simulink model "HoppingRobotModel"  (R2019b)
settings: Solver=VariableStepAuto  StartTime=0.0  StopTime=10.0  RelTol=1e-3
undefined symbols (not defined in the file): g, I1, ini_theta_1, ini_thetad_1, M2, r1, r2
settings Model: Creator=fabia  LastModifiedBy=fabia

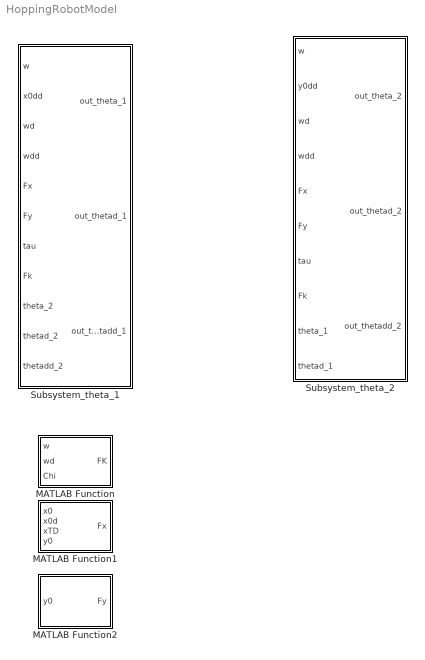
== system HoppingRobotModel ==
  MATLAB Function : MATLAB Function  TreatAsAtomicUnit=on
  MATLAB Function1 : MATLAB Function  TreatAsAtomicUnit=on
  MATLAB Function2 : MATLAB Function  TreatAsAtomicUnit=on
  Subsystem_theta_1 : Subsystem
  Subsystem_theta_2 : Subsystem

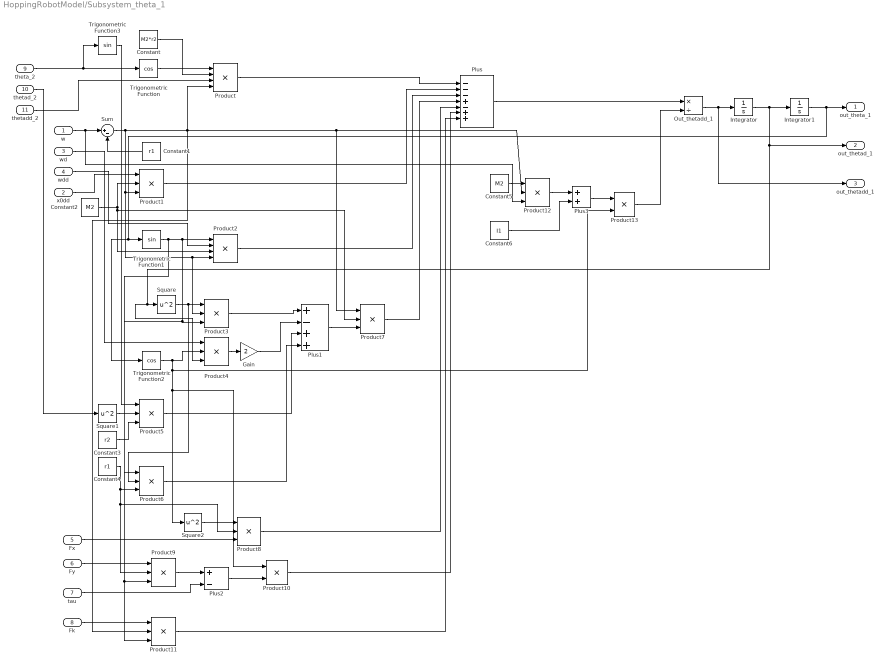
== system HoppingRobotModel/Subsystem_theta_1 ==
  w : Inport
  x0dd : Inport  Port=2
  wd : Inport  Port=3
  wdd : Inport  Port=4
  Fx : Inport  Port=5
  Fy : Inport  Port=6
  tau : Inport  Port=7
  Fk : Inport  Port=8
  theta_2 : Inport  Port=9
  thetad_2 : Inport  Port=10
  thetadd_2 : Inport  Port=11
  Constant : Constant  Value=M2*r2
  Constant1 : Constant  Value=r1
  Constant2 : Constant  Value=M2
  Constant3 : Constant  Value=r2
  Constant4 : Constant  Value=r1
  Constant5 : Constant  Value=M2
  Constant6 : Constant  Value=I1
  Gain : Gain  Gain=2
  Integrator : Integrator  InitialCondition=ini_thetad_1
  Integrator1 : Integrator  InitialCondition=ini_theta_1
  Out_thetadd_1 : Product  Inputs=*/
  Plus : Sum  Inputs=---+-++
  Plus1 : Sum  Inputs=+-++
  Plus2 : Sum  Inputs=+-
  Plus3 : Sum
  Product : Product  Inputs=4
  Product{1,3..9,11..12} (10 alike) : Product  Inputs=3
  Product10 : Product
  Product13 : Product
  Product2 : Product  Inputs=4
  Square : Math  Operator=square  SignedPower=off  SaturateOnIntegerOverflow=on
  Square1 : Math  Operator=square  SignedPower=off  SaturateOnIntegerOverflow=on
  Square2 : Math  Operator=square  SignedPower=off  SaturateOnIntegerOverflow=on
  Sum : Sum  Inputs=|+-
  Trigonometric Function : Trigonometry  Operator=cos
  Trigonometric Function1 : Trigonometry
  Trigonometric Function2 : Trigonometry  Operator=cos
  Trigonometric Function3 : Trigonometry
  out_theta_1 : Outport
  out_thetad_1 : Outport  Port=2
  out_thetadd_1 : Outport  Port=3
  wires:
  Trigonometric Function/1 -> Product/1
  Constant/1 -> Product/2
  Out_thetadd_1/1 -> out_thetadd_1/1, Integrator/1
  w/1 -> Product12/3, Sum/1
  Sum/1 -> Product2/4, Product3/2, Product1/3, Product11/2, Product12/2, Product7/1, Product/4
  x0dd/1 -> Product1/1
  Constant2/1 -> Product7/2, Product2/3, Product1/2
  Product/1 -> Plus/1
  Product1/1 -> Plus/2
  Trigonometric Function1/1 -> Product9/3, Product11/3, Product6/1, Product3/3, Product2/1
  Integrator1/1 -> Trigonometric Function2/1, Trigonometric Function1/1, out_theta_1/1
  wdd/1 -> Product2/2
  Product2/1 -> Plus/3
  Constant1/1 -> Sum/2
  Square/1 -> Product6/2, Product3/1
  Integrator/1 -> out_thetad_1/1, Product4/3, Square/1, Integrator1/1
  Product3/1 -> Plus1/1
  wd/1 -> Product4/1
  Trigonometric Function2/1 -> Product4/2, Product13/2, Product10/1, Square2/1
  Product4/1 -> Gain/1
  Gain/1 -> Plus1/2
  Trigonometric Function3/1 -> Product5/1
  Square1/1 -> Product5/2
  Constant3/1 -> Product5/3
  Product5/1 -> Plus1/3
  Constant4/1 -> Product9/2, Product8/2, Product6/3
  Product6/1 -> Plus1/4
  Plus1/1 -> Product7/3
  Product7/1 -> Plus/4
  Square2/1 -> Product8/1
  Fx/1 -> Product8/3
  Product8/1 -> Plus/5
  Fy/1 -> Product9/1
  Product9/1 -> Plus2/1
  tau/1 -> Plus2/2
  Plus2/1 -> Product10/2
  Product10/1 -> Plus/6
  Fk/1 -> Product11/1
  Product11/1 -> Plus/7
  Plus/1 -> Out_thetadd_1/1
  Constant5/1 -> Product12/1
  Product12/1 -> Plus3/1
  Constant6/1 -> Plus3/2
  Plus3/1 -> Product13/1
  Product13/1 -> Out_thetadd_1/2
  thetadd_2/1 -> Product/3
  theta_2/1 -> Trigonometric Function3/1, Trigonometric Function/1
  thetad_2/1 -> Square1/1

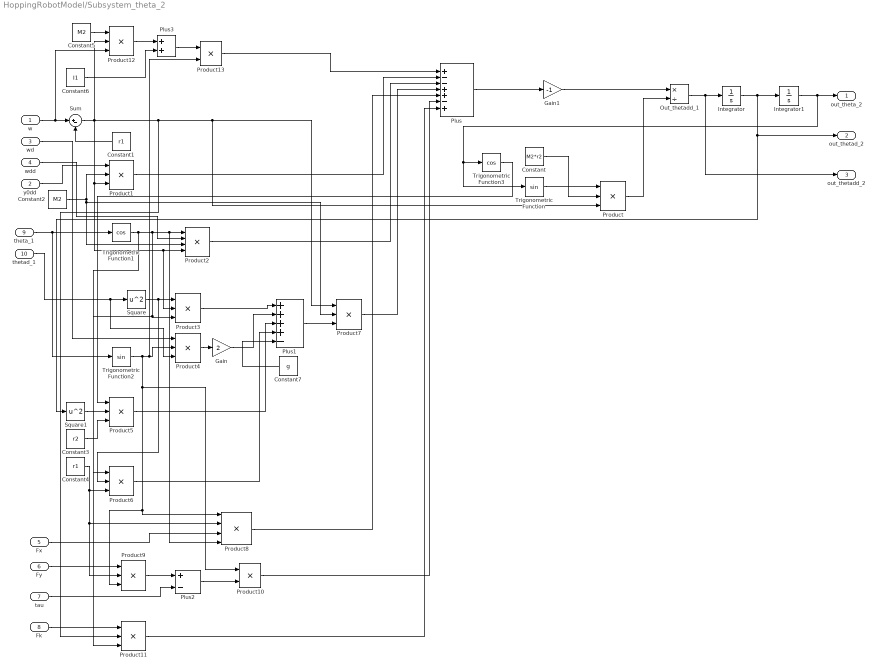
== system HoppingRobotModel/Subsystem_theta_2 ==
  w : Inport
  y0dd : Inport  Port=2
  wd : Inport  Port=3
  wdd : Inport  Port=4
  Fx : Inport  Port=5
  Fy : Inport  Port=6
  tau : Inport  Port=7
  Fk : Inport  Port=8
  theta_1 : Inport  Port=9
  thetad_1 : Inport  Port=10
  Constant : Constant  Value=M2*r2
  Constant1 : Constant  Value=r1
  Constant2 : Constant  Value=M2
  Constant3 : Constant  Value=r2
  Constant4 : Constant  Value=r1
  Constant5 : Constant  Value=M2
  Constant6 : Constant  Value=I1
  Constant7 : Constant  Value=g
  Gain : Gain  Gain=2
  Gain1 : Gain  Gain=-1
  Integrator : Integrator  InitialCondition=ini_thetad_1
  Integrator1 : Integrator  InitialCondition=ini_theta_1
  Out_thetadd_1 : Product  Inputs=*/
  Plus : Sum  Inputs=+--++-+
  Plus1 : Sum  Inputs=++++-
  Plus2 : Sum  Inputs=+-
  Plus3 : Sum
  Product{,1,3..7,9,11..12} (10 alike) : Product  Inputs=3
  Product10 : Product
  Product13 : Product
  Product2 : Product  Inputs=4
  Product8 : Product  Inputs=4
  Square : Math  Operator=square  SignedPower=off  SaturateOnIntegerOverflow=on
  Square1 : Math  Operator=square  SignedPower=off  SaturateOnIntegerOverflow=on
  Sum : Sum  Inputs=|+-
  Trigonometric Function : Trigonometry
  Trigonometric Function1 : Trigonometry  Operator=cos
  Trigonometric Function2 : Trigonometry
  Trigonometric Function3 : Trigonometry  Operator=cos
  out_theta_2 : Outport
  out_thetad_2 : Outport  Port=2
  out_thetadd_2 : Outport  Port=3
  wires:
  Out_thetadd_1/1 -> out_thetadd_2/1, Integrator/1
  w/1 -> Product12/3, Sum/1
  Sum/1 -> Product12/2, Product2/4, Product3/2, Product1/3, Product11/2, Product/3, Product7/1
  y0dd/1 -> Product1/1
  Constant2/1 -> Product7/2, Product2/3, Product1/2
  Product1/1 -> Plus/2
  Trigonometric Function1/1 -> Product8/4, Product2/1, Product6/1, Product3/3, Product11/3
  Integrator1/1 -> Trigonometric Function3/1, Trigonometric Function/1, out_theta_2/1
  wdd/1 -> Product2/2
  Product2/1 -> Plus/3
  Constant1/1 -> Sum/2
  Square/1 -> Product6/2, Product3/1
  Integrator/1 -> out_thetad_2/1, Square1/1, Integrator1/1
  Product3/1 -> Plus1/1
  wd/1 -> Product4/1
  Product4/1 -> Gain/1
  Gain/1 -> Plus1/2
  Square1/1 -> Product5/2
  Constant3/1 -> Product5/3
  Product5/1 -> Plus1/3
  Constant4/1 -> Product9/2, Product8/2, Product6/3
  Product6/1 -> Plus1/4
  Plus1/1 -> Product7/3
  Product7/1 -> Plus/4
  Trigonometric Function2/1 -> Product13/2, Product4/2, Product9/3, Product8/1, Product10/1
  Fx/1 -> Product8/3
  Product8/1 -> Plus/5
  Fy/1 -> Product9/1
  Product9/1 -> Plus2/1
  tau/1 -> Plus2/2
  Plus2/1 -> Product10/2
  Product10/1 -> Plus/6
  Fk/1 -> Product11/1
  Product11/1 -> Plus/7
  Constant5/1 -> Product12/1
  Product12/1 -> Plus3/1
  Plus3/1 -> Product13/1
  Constant/1 -> Product/2
  Constant6/1 -> Plus3/2
  theta_1/1 -> Trigonometric Function2/1, Trigonometric Function1/1
  thetad_1/1 -> Product4/3, Square/1
  Product13/1 -> Plus/1
  Trigonometric Function/1 -> Product/1
  Trigonometric Function3/1 -> Product5/1
  Constant7/1 -> Plus1/5
  Plus/1 -> Gain1/1
  Gain1/1 -> Out_thetadd_1/1
  Product/1 -> Out_thetadd_1/2

== matlab function HoppingRobotModel/MATLAB Function1 ==
  data: x0 input; Fx output; x0d input; xTD input; y0 input
function Fx = fcn(x0,x0d,xTD,y0)
if y0<0
   Fx = -KG*(x0-xTD)-(BG*x0d);
else
    Fx=0;
end

== matlab function HoppingRobotModel/MATLAB Function ==
  data: w input; FK output; wd input; Chi input
function FK = fcn(w,wd,Chi)
if (k0-w+Chi)>0
   FK = KL*(k0-w+Chi);
else
    FK=KL2*(k0-w+Chi)-(BL2*wd);
end

== matlab function HoppingRobotModel/MATLAB Function2 ==
  data: Fy output; y0 input
function Fy = fcn(y0)
if y0<0
   Fy = (-KG*y0)-(BG*y0);
else
    Fy=0;
end
